simulink library "FUSA_ACTMON"  (R2024b)
settings: Solver=VariableStepAuto  StartTime=0.0  StopTime=10.0  RelTol=1e-3
undefined symbols (not defined in the file or in its folder): FUSA_ACTMON_p_AngDmpErrThr_deg, FUSA_ACTMON_p_NConfirm_na
libraries: VUT_lib x1
settings Model: Creator=jmbsp  LastModifiedBy=jmbsp

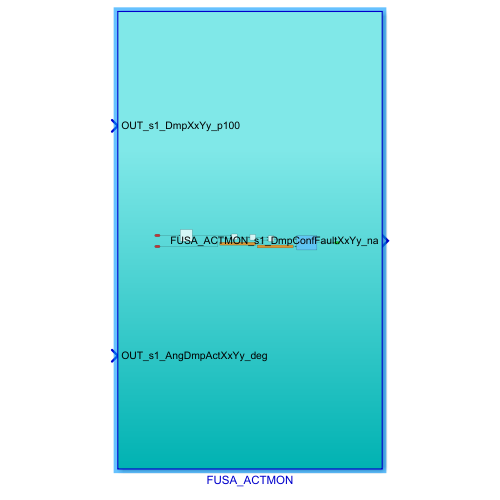
[thumbnail: Simulink's stored preview of the top-level diagram]
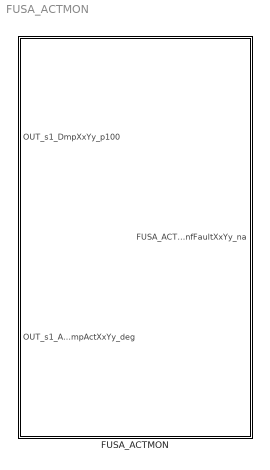
== system FUSA_ACTMON ==
  FUSA_ACTMON : Subsystem

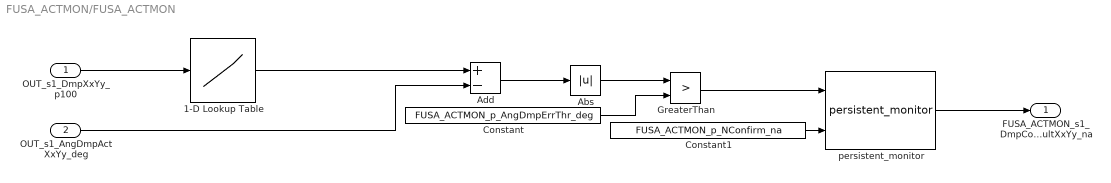
== system FUSA_ACTMON/FUSA_ACTMON ==
  OUT_s1_DmpXxYy_p100 : Inport
  OUT_s1_AngDmpActXxYy_deg : Inport  Port=2
  1-D Lookup Table : Lookup_n-D  NumberOfTableDimensions=1  BreakpointsForDimension1=[0 10 20 30 40 50 60 70 80 90 100]  Table=[0 5 10 15 20 25 30 35 40 45 50]  InternalRulePriority=Speed  RndMeth=Simplest
  Abs : Abs  SaturateOnIntegerOverflow=off
  Add : Sum  Inputs=+-
  Constant : Constant  Value=FUSA_ACTMON_p_AngDmpErrThr_deg
  Constant1 : Constant  Value=FUSA_ACTMON_p_NConfirm_na
  GreaterThan : RelationalOperator  Operator=>  OutDataTypeStr=boolean  RndMeth=Simplest  InputSameDT=off
  persistent_monitor : VUT_lib/persistent_monitor  SystemSampleTime=-1  VariantActivationTime=update diagram  AllowFlexibleInterface=on  Latency=0  AutoFrameSizeCalculation=off
  FUSA_ACTMON_s1_DmpConfFaultXxYy_na : Outport
  wires:
  OUT_s1_AngDmpActXxYy_deg/1 -> Add/2
  Add/1 -> Abs/1
  Abs/1 -> GreaterThan/1
  Constant/1 -> GreaterThan/2
  OUT_s1_DmpXxYy_p100/1 -> 1-D Lookup Table/1
  1-D Lookup Table/1 -> Add/1
  GreaterThan/1 -> persistent_monitor/1
  persistent_monitor/1 -> FUSA_ACTMON_s1_DmpConfFaultXxYy_na/1
  Constant1/1 -> persistent_monitor/2
